simulink model "Zencar_rpo_2020_HIL_simulinkModel_PrebijaciStroj"  (R2020a)
settings: Solver=FixedStepAuto  StartTime=0.0  StopTime=150  FixedStep=1e-5  RelTol=1e-3
values from neighbouring files (symbols this model uses):
  b = 0.0002    [Zencar_rpo_2020_HIL_paramDef_PrebijaciStroj.m]
  cfi = 0.0137    [Zencar_rpo_2020_HIL_paramDef_PrebijaciStroj.m]
  g = 9.81    [Zencar_rpo_2020_HIL_paramDef_PrebijaciStroj.m]
  GR_overall = GR_rot*GR_transl    (= 0.000943396226415)    [Zencar_rpo_2020_HIL_paramDef_PrebijaciStroj.m]
  GR_rot = 1/53    (= 0.0188679245283)    [Zencar_rpo_2020_HIL_paramDef_PrebijaciStroj.m]
  GR_transl = 0.05    [Zencar_rpo_2020_HIL_paramDef_PrebijaciStroj.m]
  hal_maxi = 100    [Zencar_rpo_2020_HIL_paramDef_PrebijaciStroj.m]
  hal_maxv = 5    [Zencar_rpo_2020_HIL_paramDef_PrebijaciStroj.m]
  hal_zerov = 2.5    [Zencar_rpo_2020_HIL_paramDef_PrebijaciStroj.m]
  initial_pos = 0.25    [Zencar_rpo_2020_HIL_paramDef_PrebijaciStroj.m]
  J = J_motor+J_gearbox+J_endgear_and_press    (= 8.64998220007e-06)    [Zencar_rpo_2020_HIL_paramDef_PrebijaciStroj.m]
  K = k    [Zencar_rpo_2020_HIL_paramDef_PrebijaciStroj.m]
  La = 0.016e-3    (= 1.6e-05)    [Zencar_rpo_2020_HIL_paramDef_PrebijaciStroj.m]
  m_sys = 5    [Zencar_rpo_2020_HIL_paramDef_PrebijaciStroj.m]
  Nbar = Nu + K*Nx    [Zencar_rpo_2020_HIL_paramDef_PrebijaciStroj.m]
  Ra = 0.102    [Zencar_rpo_2020_HIL_paramDef_PrebijaciStroj.m]
  rot_enc_ppr = 2048    [Zencar_rpo_2020_HIL_paramDef_PrebijaciStroj.m]
  stroke = 0.3    [Zencar_rpo_2020_HIL_paramDef_PrebijaciStroj.m]
  Umax = 24    [Zencar_rpo_2020_HIL_paramDef_PrebijaciStroj.m]
settings Model: Creator=Palo  LastModifiedBy=Palo

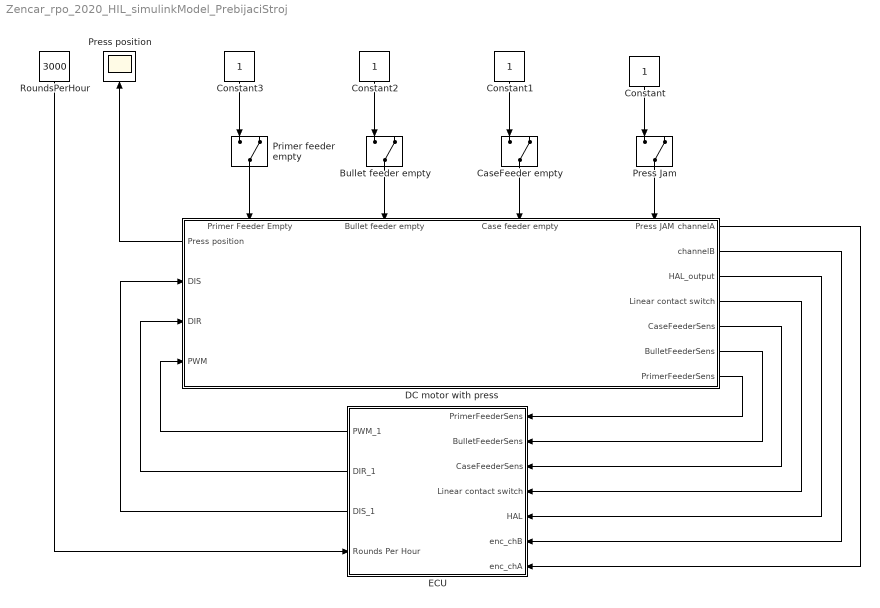
== system Zencar_rpo_2020_HIL_simulinkModel_PrebijaciStroj ==
  Bullet feeder empty : ManualSwitch  CurrentSetting=0
  CaseFeeder empty : ManualSwitch  CurrentSetting=0
  Constant{,1..3} (4 alike) : Constant
  DC motor with press : Subsystem
      settings: PortSchema="{\"entries\":[{\"content\":{\"sides\":[{\"content\":{\"connectorIds\":[\"Out8\",\"In1\",\"In2\",\"In3\"]},\"type\":\"ConnectorPlacement.EquallySpacedRectSide\",\"uuid\":\"44aa01d9-a270-4b10-8569-0796e281ce1b\"},{\"content\":{\"connectorIds\":[\"Out1\",\"Out2\",\"Out3\",\"Out4\",\"Out5\",\"Out6\",\"Out7\"],\"side\":\"RIGHT\"},\"type\":\"ConnectorPlacement.EquallySpacedRectSide\",\"uuid\":\"c8e5899d-1334-4fa1-8867-c03f8e90729c\"},{\"content\":{\"connectorIds\":[\"In4\",\"In5\",\"In6\",\"In7\"],\"side\":\"TOP\"},\"type\":\"ConnectorPlacement.EquallySpacedRectSide\",\"uuid\":\"b199ad83-4d3f-426f-a24f-893a662e75fe\"}]},\"type\":\"ConnectorPlacement.EquallySpacedConnector\",\"uuid\":\"598d06f8-804a-47b4-ba62-695d707896bf\"}],\"packageUris\":[\"http://schema.mathworks.com/mf0/Connector/19700101\"],\"version\":\"1.0\"}"
  ECU : Subsystem
      settings: PortSchema="{\"entries\":[{\"content\":{\"sides\":[{\"content\":{\"connectorIds\":[\"In1\",\"In2\",\"In3\",\"In4\",\"In5\",\"In6\",\"In7\"]},\"type\":\"ConnectorPlacement.EquallySpacedRectSide\",\"uuid\":\"89d60bc3-cc9c-43a7-ae0f-bebf81c284df\"},{\"content\":{\"connectorIds\":[\"Out1\",\"Out2\",\"Out3\",\"In8\"],\"side\":\"RIGHT\"},\"type\":\"ConnectorPlacement.EquallySpacedRectSide\",\"uuid\":\"e25504cb-4fdc-4ec0-83be-a621ed95c836\"},{\"content\":{\"connectorIds\":[],\"side\":\"TOP\"},\"type\":\"ConnectorPlacement.EquallySpacedRectSide\",\"uuid\":\"3fb693ce-24d4-4cc1-a1ce-0deb39646084\"}]},\"type\":\"ConnectorPlacement.EquallySpacedConnector\",\"uuid\":\"2bc13cae-35da-4195-ba30-c3443b14a144\"}],\"packageUris\":[\"http://schema.mathworks.com/mf0/Connector/19700101\"],\"version\":\"1.0\"}"
  Press Jam : ManualSwitch  CurrentSetting=0
  Press position : Scope
  Primer feeder empty : ManualSwitch  CurrentSetting=0
  RoundsPerHour : Constant  Value=3000
  wires:
  DC motor with press/1(channelA) -> ECU/7(enc_chA)
  DC motor with press/2(channelB) -> ECU/6(enc_chB)
  DC motor with press/3(HAL_output) -> ECU/5(HAL)
  ECU/1(PWM_1) -> DC motor with press/3(PWM)
  ECU/2(DIR_1) -> DC motor with press/2(DIR)
  ECU/3(DIS_1) -> DC motor with press/1(DIS)
  DC motor with press/4(Linear contact switch) -> ECU/4(Linear contact switch)
  Constant/1 -> Press Jam/1
  CaseFeeder empty/1 -> DC motor with press/6(Case feeder empty)
  Constant1/1 -> CaseFeeder empty/1
  Constant2/1 -> Bullet feeder empty/1
  DC motor with press/6(BulletFeederSens) -> ECU/2(BulletFeederSens)
  DC motor with press/5(CaseFeederSens) -> ECU/3(CaseFeederSens)
  Primer feeder empty/1 -> DC motor with press/4(Primer Feeder Empty)
  Constant3/1 -> Primer feeder empty/1
  DC motor with press/7(PrimerFeederSens) -> ECU/1(PrimerFeederSens)
  DC motor with press/8(Press position) -> Press position/1
  RoundsPerHour/1 -> ECU/8(Rounds Per Hour)
  Bullet feeder empty/1 -> DC motor with press/5(Bullet feeder empty)
  Press Jam/1 -> DC motor with press/7(Press JAM)

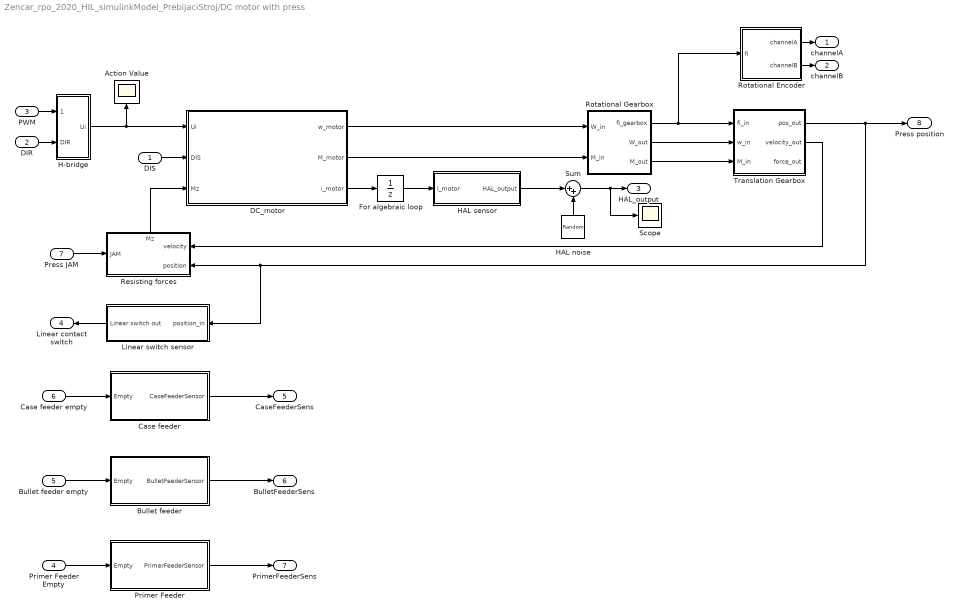
== system Zencar_rpo_2020_HIL_simulinkModel_PrebijaciStroj/DC motor with press ==
  DIS : Inport
  DIR : Inport  Port=2
  PWM : Inport  Port=3
  Primer Feeder Empty : Inport  Port=4
  Bullet feeder empty : Inport  Port=5
  Case feeder empty : Inport  Port=6
  Press JAM : Inport  Port=7
  Action Value : Scope
  Bullet feeder : Subsystem
  Case feeder : Subsystem
  DC_motor : Subsystem
  For algebraic loop : UnitDelay  SampleTime=-1  HasFrameUpgradeWarning=on
  H-bridge : Subsystem
  HAL noise : RandomNumber  Variance=3.3/10000  SampleTime=0.1
  HAL sensor : Subsystem
  Linear switch sensor : Subsystem
  Primer Feeder : Subsystem
  Resisting forces : Subsystem
      settings: PortSchema="{\"entries\":[{\"content\":{\"sides\":[{\"content\":{\"connectorIds\":[\"In1\"]},\"type\":\"ConnectorPlacement.EquallySpacedRectSide\",\"uuid\":\"f66e595a-d546-4368-bb4f-170145c9d05d\"},{\"content\":{\"connectorIds\":[\"In2\",\"In3\"],\"side\":\"RIGHT\"},\"type\":\"ConnectorPlacement.EquallySpacedRectSide\",\"uuid\":\"f401b9ee-f172-4854-b1a2-c293cdbafb20\"},{\"content\":{\"connectorIds\":[\"Out1\"],\"side\":\"TOP\"},\"type\":\"ConnectorPlacement.EquallySpacedRectSide\",\"uuid\":\"bb4b329b-5312-4992-9255-fed05c1ebbda\"}]},\"type\":\"ConnectorPlacement.EquallySpacedConnector\",\"uuid\":\"f4d49964-271c-4275-b048-9eeda0ea6065\"}],\"packageUris\":[\"http://schema.mathworks.com/mf0/Connector/19700101\"],\"version\":\"1.0\"}"
  Rotational Encoder : Subsystem
  Rotational Gearbox : Subsystem
  Scope : Scope
  Sum : Sum  Inputs=|++
  Translation Gearbox : Subsystem
  channelA : Outport
  channelB : Outport  Port=2
  HAL_output : Outport  Port=3
  Linear contact switch : Outport  Port=4
  CaseFeederSens : Outport  Port=5
  BulletFeederSens : Outport  Port=6
  PrimerFeederSens : Outport  Port=7
  Press position : Outport  Port=8
  wires:
  DC_motor/1(w_motor) -> Rotational Gearbox/1(W_in)
  DIR/1 -> H-bridge/2(DIR)
  Rotational Gearbox/2(W_out) -> Translation Gearbox/2(w_in)
  DC_motor/2(M_motor) -> Rotational Gearbox/2(M_in)
  H-bridge/1(Ui) -> DC_motor/1(Ui), Action Value/1
  Rotational Gearbox/3(M_out) -> Translation Gearbox/3(M_in)
  Rotational Encoder/2(channelB) -> channelB/1
  Rotational Encoder/1(channelA) -> channelA/1
  PWM/1 -> H-bridge/1(PWM)
  DC_motor/3(i_motor) -> For algebraic loop/1
  Rotational Gearbox/1(fi_gearbox) -> Rotational Encoder/1(fi), Translation Gearbox/1(fi_in)
  DIS/1 -> DC_motor/2(DIS)
  Translation Gearbox/1(pos_out) -> Press position/1, Resisting forces/3(position), Linear switch sensor/1(position_in)
  Translation Gearbox/2(velocity_out) -> Resisting forces/2(velocity)
  Linear switch sensor/1(Linear switch out) -> Linear contact switch/1
  Press JAM/1 -> Resisting forces/1(JAM)
  Case feeder empty/1 -> Case feeder/1(Empty)
  Bullet feeder empty/1 -> Bullet feeder/1(Empty)
  Bullet feeder/1(BulletFeederSensor) -> BulletFeederSens/1
  Case feeder/1(CaseFeederSensor) -> CaseFeederSens/1
  Primer Feeder/1(PrimerFeederSensor) -> PrimerFeederSens/1
  Primer Feeder Empty/1 -> Primer Feeder/1(Empty)
  For algebraic loop/1 -> HAL sensor/1(I_motor)
  HAL sensor/1(HAL_output) -> Sum/1
  Sum/1 -> Scope/1, HAL_output/1
  HAL noise/1 -> Sum/2
  Resisting forces/1(Mz) -> DC_motor/3(Mz)

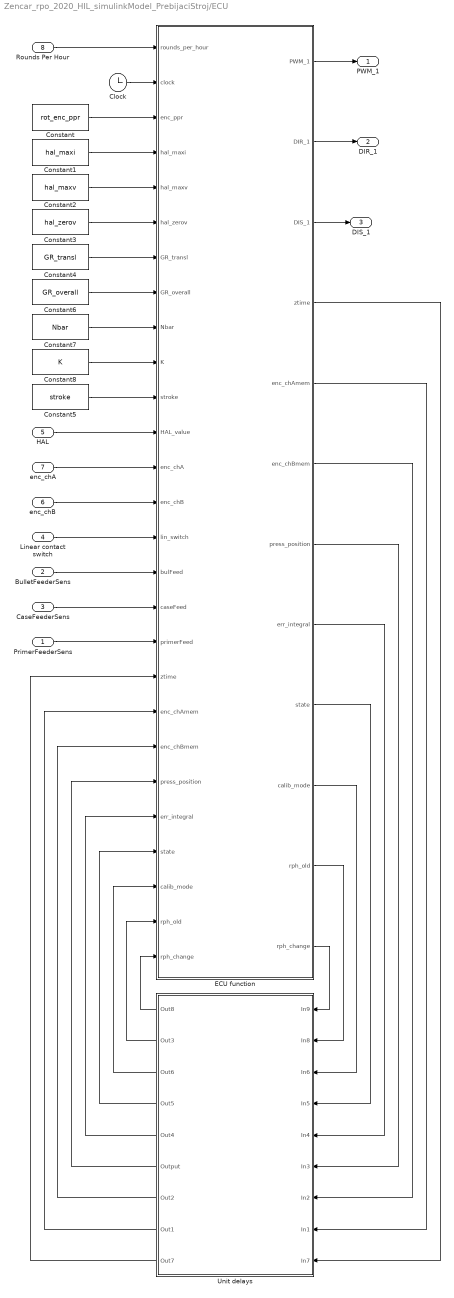
== system Zencar_rpo_2020_HIL_simulinkModel_PrebijaciStroj/ECU ==
  PrimerFeederSens : Inport
  BulletFeederSens : Inport  Port=2
  CaseFeederSens : Inport  Port=3
  Linear contact switch : Inport  Port=4
  HAL : Inport  Port=5
  enc_chB : Inport  Port=6
  enc_chA : Inport  Port=7
  Rounds Per Hour : Inport  Port=8
  Clock : Clock
  Constant : Constant  Value=rot_enc_ppr
  Constant1 : Constant  Value=hal_maxi
  Constant2 : Constant  Value=hal_maxv
  Constant3 : Constant  Value=hal_zerov
  Constant4 : Constant  Value=GR_transl
  Constant5 : Constant  Value=stroke
  Constant6 : Constant  Value=GR_overall
  Constant7 : Constant  Value=Nbar
  Constant8 : Constant  Value=K  VectorParams1D=off
  ECU function : MATLAB Function  TreatAsAtomicUnit=on
  Unit delays : Subsystem
  PWM_1 : Outport
  DIR_1 : Outport  Port=2
  DIS_1 : Outport  Port=3
  wires:
  enc_chA/1 -> ECU function/13(enc_chA)
  enc_chB/1 -> ECU function/14(enc_chB)
  ECU function/1(PWM_1) -> PWM_1/1
  ECU function/2(DIR_1) -> DIR_1/1
  Constant/1 -> ECU function/3(enc_ppr)
  HAL/1 -> ECU function/12(HAL_value)
  Constant1/1 -> ECU function/4(hal_maxi)
  Constant3/1 -> ECU function/6(hal_zerov)
  Constant2/1 -> ECU function/5(hal_maxv)
  ECU function/3(DIS_1) -> DIS_1/1
  Constant4/1 -> ECU function/7(GR_transl)
  Linear contact switch/1 -> ECU function/15(lin_switch)
  ECU function/5(enc_chAmem) -> Unit delays/8(In1)
  ECU function/6(enc_chBmem) -> Unit delays/7(In2)
  ECU function/8(err_integral) -> Unit delays/5(In4)
  Unit delays/8(Out1) -> ECU function/20("enc_chAmem ")
  Unit delays/7(Out2) -> ECU function/21("enc_chBmem ")
  Unit delays/6(Output) -> ECU function/22("press_position ")
  Unit delays/5(Out4) -> ECU function/23("err_integral ")
  ECU function/9(state) -> Unit delays/4(In5)
  ECU function/10(calib_mode) -> Unit delays/3(In6)
  Unit delays/4(Out5) -> ECU function/24("state ")
  Unit delays/3(Out6) -> ECU function/25("calib_mode ")
  Constant5/1 -> ECU function/11(stroke)
  Clock/1 -> ECU function/2(clock)
  Unit delays/9(Out7) -> ECU function/19("ztime ")
  ECU function/4(ztime) -> Unit delays/9(In7)
  BulletFeederSens/1 -> ECU function/16(bulFeed)
  CaseFeederSens/1 -> ECU function/17(caseFeed)
  PrimerFeederSens/1 -> ECU function/18(primerFeed)
  Unit delays/2(Out3) -> ECU function/26("rph_old ")
  ECU function/11(rph_old) -> Unit delays/2(In8)
  Unit delays/1(Out8) -> ECU function/27("rph_change ")
  ECU function/12(rph_change) -> Unit delays/1(In9)
  Rounds Per Hour/1 -> ECU function/1(rounds_per_hour)
  ECU function/7(press_position) -> Unit delays/6(In3)
  Constant6/1 -> ECU function/8(GR_overall)
  Constant7/1 -> ECU function/9(Nbar)
  Constant8/1 -> ECU function/10(K)

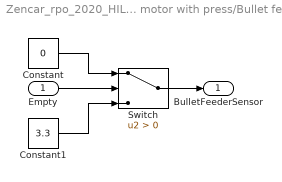
== system Zencar_rpo_2020_HIL_simulinkModel_PrebijaciStroj/DC motor with press/Bullet feeder ==
  Empty : Inport
  Constant : Constant  Value=0
  Constant1 : Constant  Value=3.3
  Switch : Switch  Criteria=u2 > Threshold
  BulletFeederSensor : Outport
  wires:
  Switch/1 -> BulletFeederSensor/1
  Constant1/1 -> Switch/3
  Constant/1 -> Switch/1
  Empty/1 -> Switch/2

== system Zencar_rpo_2020_HIL_simulinkModel_PrebijaciStroj/DC motor with press/Case feeder ==
  Empty : Inport
  Constant : Constant  Value=0
  Constant1 : Constant  Value=3.3
  Switch : Switch  Criteria=u2 > Threshold
  CaseFeederSensor : Outport
  wires:
  Empty/1 -> Switch/2
  Constant/1 -> Switch/1
  Constant1/1 -> Switch/3
  Switch/1 -> CaseFeederSensor/1

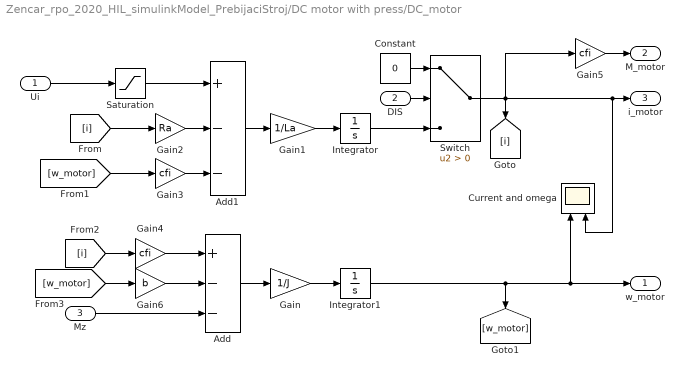
== system Zencar_rpo_2020_HIL_simulinkModel_PrebijaciStroj/DC motor with press/DC_motor ==
  Ui : Inport
  DIS : Inport  Port=2
  Mz : Inport  Port=3
  Add : Sum  Inputs=+--
  Add1 : Sum  Inputs=+--
  Constant : Constant  Value=0
  Current and omega : Scope  NumInputPorts=2
  Gain : Gain  Gain=1/J
  Gain1 : Gain  Gain=1/La
  Gain2 : Gain  Gain=Ra
  Gain3 : Gain  Gain=cfi
  Gain4 : Gain  Gain=cfi
  Gain5 : Gain  Gain=cfi
  Gain6 : Gain  Gain=b
  Integrator : Integrator
  Integrator1 : Integrator
  Saturation : Saturate  UpperLimit=Umax  LowerLimit=-Umax
  Switch : Switch  Criteria=u2 > Threshold
  w_motor : Outport
  M_motor : Outport  Port=2
  i_motor : Outport  Port=3
  wires:
  Add/1 -> Gain/1
  Gain/1 -> Integrator1/1
  Gain1/1 -> Integrator/1
  Add1/1 -> Gain1/1
  Gain2/1 -> Add1/2
  [i] -> Gain2/1
  [i] -> Gain4/1
  Gain3/1 -> Add1/3
  [w_motor] -> Gain3/1
  Gain4/1 -> Add/1
  Ui/1 -> Saturation/1
  Saturation/1 -> Add1/1
  Gain5/1 -> M_motor/1
  Integrator/1 -> Switch/3
  Switch/1 -> i_motor/1, Current and omega/2, Gain5/1, [i]
  DIS/1 -> Switch/2
  Constant/1 -> Switch/1
  Integrator1/1 -> Current and omega/1, w_motor/1, [w_motor]
  Mz/1 -> Add/3
  [w_motor] -> Gain6/1
  Gain6/1 -> Add/2

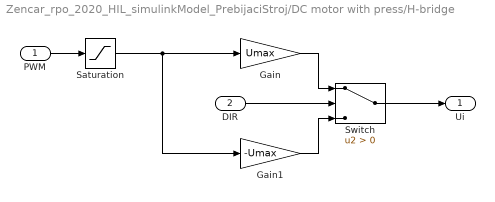
== system Zencar_rpo_2020_HIL_simulinkModel_PrebijaciStroj/DC motor with press/H-bridge ==
  PWM : Inport
  DIR : Inport  Port=2
  Gain : Gain  Gain=Umax
  Gain1 : Gain  Gain=-Umax
  Saturation : Saturate  UpperLimit=1  LowerLimit=0
  Switch : Switch  Criteria=u2 > Threshold
  Ui : Outport
  wires:
  DIR/1 -> Switch/2
  Gain/1 -> Switch/1
  PWM/1 -> Saturation/1
  Saturation/1 -> Gain1/1, Gain/1
  Gain1/1 -> Switch/3
  Switch/1 -> Ui/1

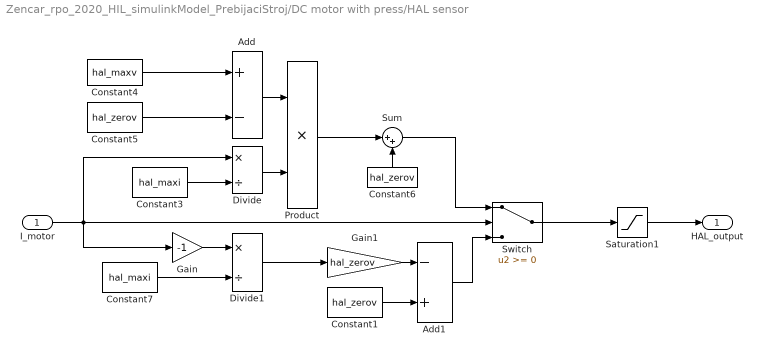
== system Zencar_rpo_2020_HIL_simulinkModel_PrebijaciStroj/DC motor with press/HAL sensor ==
  I_motor : Inport
  Add : Sum  Inputs=+-
  Add1 : Sum  Inputs=-+
  Constant1 : Constant  Value=hal_zerov
  Constant3 : Constant  Value=hal_maxi
  Constant4 : Constant  Value=hal_maxv
  Constant5 : Constant  Value=hal_zerov
  Constant6 : Constant  Value=hal_zerov
  Constant7 : Constant  Value=hal_maxi
  Divide : Product  Inputs=*/
  Divide1 : Product  Inputs=*/
  Gain : Gain  Gain=-1
  Gain1 : Gain  Gain=hal_zerov
  Product : Product
  Saturation1 : Saturate  UpperLimit=4.5  LowerLimit=0.5
  Sum : Sum  Inputs=|++
  Switch : Switch
  HAL_output : Outport
  wires:
  Constant4/1 -> Add/1
  Constant5/1 -> Add/2
  Add/1 -> Product/1
  Divide/1 -> Product/2
  Constant3/1 -> Divide/2
  Product/1 -> Sum/1
  Sum/1 -> Switch/1
  Constant6/1 -> Sum/2
  Gain/1 -> Divide1/1
  Constant7/1 -> Divide1/2
  Divide1/1 -> Gain1/1
  I_motor/1 -> Gain/1, Switch/2, Divide/1
  Gain1/1 -> Add1/1
  Add1/1 -> Switch/3
  Constant1/1 -> Add1/2
  Switch/1 -> Saturation1/1
  Saturation1/1 -> HAL_output/1

== system Zencar_rpo_2020_HIL_simulinkModel_PrebijaciStroj/DC motor with press/Linear switch sensor ==
  position_in : Inport
  Constant : Constant  Value=0
  Constant1 : Constant
  Switch : Switch  Threshold=stroke*0.25
  Linear switch out : Outport
  wires:
  position_in/1 -> Switch/2
  Constant/1 -> Switch/1
  Constant1/1 -> Switch/3
  Switch/1 -> Linear switch out/1

== system Zencar_rpo_2020_HIL_simulinkModel_PrebijaciStroj/DC motor with press/Primer Feeder ==
  Empty : Inport
  Constant : Constant  Value=0
  Constant1 : Constant  Value=3.3
  Switch : Switch  Criteria=u2 > Threshold
  PrimerFeederSensor : Outport
  wires:
  Switch/1 -> PrimerFeederSensor/1
  Constant1/1 -> Switch/3
  Constant/1 -> Switch/1
  Empty/1 -> Switch/2

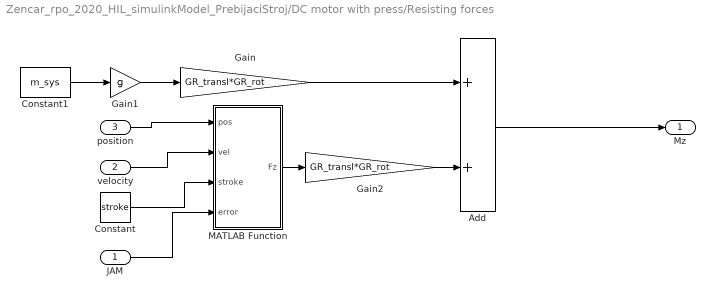
== system Zencar_rpo_2020_HIL_simulinkModel_PrebijaciStroj/DC motor with press/Resisting forces ==
  JAM : Inport
  velocity : Inport  Port=2
  position : Inport  Port=3
  Add : Sum
  Constant : Constant  Value=stroke
  Constant1 : Constant  Value=m_sys
  Gain : Gain  Gain=GR_transl*GR_rot
  Gain1 : Gain  Gain=g
  Gain2 : Gain  Gain=GR_transl*GR_rot
  MATLAB Function : MATLAB Function  TreatAsAtomicUnit=on
  Mz : Outport
  wires:
  Gain1/1 -> Gain/1
  Gain/1 -> Add/1
  Constant1/1 -> Gain1/1
  MATLAB Function/1(Fz) -> Gain2/1
  position/1 -> MATLAB Function/1(pos)
  velocity/1 -> MATLAB Function/2(vel)
  Constant/1 -> MATLAB Function/3(stroke)
  Add/1 -> Mz/1
  JAM/1 -> MATLAB Function/4(error)
  Gain2/1 -> Add/2

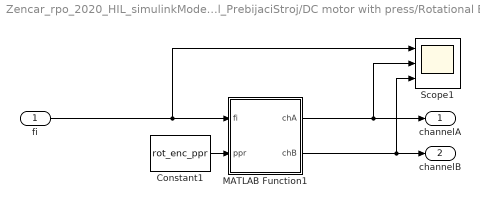
== system Zencar_rpo_2020_HIL_simulinkModel_PrebijaciStroj/DC motor with press/Rotational Encoder ==
  fi : Inport
  Constant1 : Constant  Value=rot_enc_ppr
  MATLAB Function1 : MATLAB Function  TreatAsAtomicUnit=on
  Scope1 : Scope  NumInputPorts=3
  channelA : Outport
  channelB : Outport  Port=2
  wires:
  MATLAB Function1/2(chB) -> channelB/1, Scope1/3
  Constant1/1 -> MATLAB Function1/2(ppr)
  MATLAB Function1/1(chA) -> channelA/1, Scope1/2
  fi/1 -> Scope1/1, MATLAB Function1/1(fi)

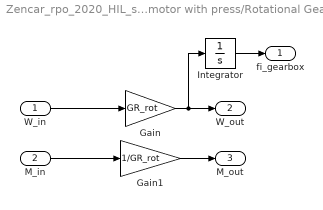
== system Zencar_rpo_2020_HIL_simulinkModel_PrebijaciStroj/DC motor with press/Rotational Gearbox ==
  W_in : Inport
  M_in : Inport  Port=2
  Gain : Gain  Gain=GR_rot
  Gain1 : Gain  Gain=1/GR_rot
  Integrator : Integrator  InitialCondition=initial_pos/GR_transl
  fi_gearbox : Outport
  W_out : Outport  Port=2
  M_out : Outport  Port=3
  wires:
  W_in/1 -> Gain/1
  M_in/1 -> Gain1/1
  Gain/1 -> Integrator/1, W_out/1
  Gain1/1 -> M_out/1
  Integrator/1 -> fi_gearbox/1

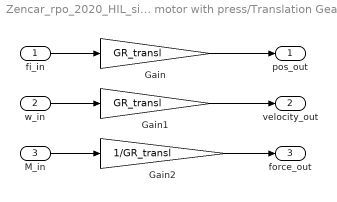
== system Zencar_rpo_2020_HIL_simulinkModel_PrebijaciStroj/DC motor with press/Translation Gearbox ==
  fi_in : Inport
  w_in : Inport  Port=2
  M_in : Inport  Port=3
  Gain : Gain  Gain=GR_transl
  Gain1 : Gain  Gain=GR_transl
  Gain2 : Gain  Gain=1/GR_transl
  pos_out : Outport
  velocity_out : Outport  Port=2
  force_out : Outport  Port=3
  wires:
  fi_in/1 -> Gain/1
  Gain/1 -> pos_out/1
  Gain1/1 -> velocity_out/1
  w_in/1 -> Gain1/1
  M_in/1 -> Gain2/1
  Gain2/1 -> force_out/1

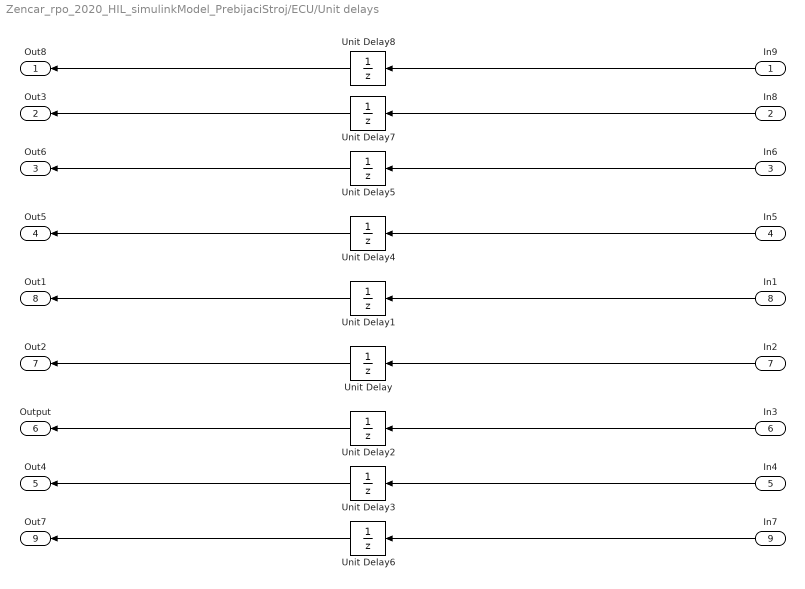
== system Zencar_rpo_2020_HIL_simulinkModel_PrebijaciStroj/ECU/Unit delays ==
  In9 : Inport
  In8 : Inport  Port=2
  In6 : Inport  Port=3
  In5 : Inport  Port=4
  In4 : Inport  Port=5
  In3 : Inport  Port=6
  In2 : Inport  Port=7
  In1 : Inport  Port=8
  In7 : Inport  Port=9
  Unit Delay{,1..8} (9 alike) : UnitDelay  SampleTime=-1  HasFrameUpgradeWarning=on
  Out8 : Outport
  Out3 : Outport  Port=2
  Out6 : Outport  Port=3
  Out5 : Outport  Port=4
  Out4 : Outport  Port=5
  Output : Outport  Port=6
  Out2 : Outport  Port=7
  Out1 : Outport  Port=8
  Out7 : Outport  Port=9
  wires:
  Unit Delay/1 -> Out2/1
  Unit Delay3/1 -> Out4/1
  Unit Delay2/1 -> Output/1
  In4/1 -> Unit Delay3/1
  In2/1 -> Unit Delay/1
  In3/1 -> Unit Delay2/1
  Unit Delay1/1 -> Out1/1
  In1/1 -> Unit Delay1/1
  In5/1 -> Unit Delay4/1
  Unit Delay5/1 -> Out6/1
  In6/1 -> Unit Delay5/1
  Unit Delay4/1 -> Out5/1
  In7/1 -> Unit Delay6/1
  Unit Delay6/1 -> Out7/1
  In8/1 -> Unit Delay7/1
  Unit Delay7/1 -> Out3/1
  In9/1 -> Unit Delay8/1
  Unit Delay8/1 -> Out8/1

== matlab function Zencar_rpo_2020_HIL_simulinkModel_PrebijaciStroj/DC motor with press/Rotational Encoder/MATLAB Function1 ==
  data: fi input; chA output; ppr input; chB output
function [chA,chB] = fcn(fi,ppr)

%clockwise direction - channel B before channel A
%anticlockwise direction - channel A before channel B

per=2*pi/ppr;%period
hper=per/2;%half period
qper=per/4;%quarter period

%channel A
zeroedFi=fi - (floor(fi/per)*per);
chA=floor(zeroedFi/hper);


%channel B
zeroedFi=fi - (floor(fi/per)*per) - qper;
if(zeroedFi<=hper &  zeroedFi>0)
    chB=1;
else
    chB=0;
end













% if(zeroedFi<=hper)
%     chA=0;
% else
%     chA=1;
% end

== matlab function Zencar_rpo_2020_HIL_simulinkModel_PrebijaciStroj/DC motor with press/Resisting forces/MATLAB Function ==
  data: pos input; Fz output; vel input; stroke input; error input
function Fz = fcn(pos,vel,stroke,error)
Fz=0;
if(vel>=0)
    if(pos > stroke*0.8)
       Fz=300; 
    else
        Fz=0;
    end
    
    if(error==1 & pos>stroke*0.9)
        Fz=15000;
    end 
    
    if(pos>stroke+0.01)
        Fz=15000;
    end
end
if(vel<0)
    if(pos<stroke*0.1)
        Fz=-150;
    else
        Fz=0;
    end
    
    if(pos>stroke*0.8)
        Fz=-150;
    end
    
    if(pos<-0.01)
        Fz=-9000;
    end
end

== matlab function Zencar_rpo_2020_HIL_simulinkModel_PrebijaciStroj/ECU/ECU function ==
  data: PWM_1 output; DIR_1 output; DIS_1 output; ztime output; enc_chAmem output; enc_chBmem output; press_position output; rounds_per_hour input; clock input; enc_ppr input; hal_maxi input; hal_maxv input; hal_zerov input; GR_transl input; GR_overall input; Nbar input; K input; stroke input; HAL_value input; enc_chA input; enc_chB input; lin_switch input; bulFeed input; caseFeed input; primerFeed input; ztime input; enc_chAmem input; enc_chBmem input; press_position input; err_integral input; err_integral output; state input; state output; calib_mode input; calib_mode output; rph_old output; rph_old input; rph_change output; rph_change input
function [PWM_1,DIR_1,DIS_1,ztime, enc_chAmem,enc_chBmem,press_position,err_integral,state, calib_mode, rph_old, rph_change] = fcn(rounds_per_hour, clock, enc_ppr,hal_maxi,hal_maxv,hal_zerov,GR_transl,GR_overall, Nbar, K, stroke, HAL_value,enc_chA,enc_chB,lin_switch,bulFeed, caseFeed, primerFeed, ztime, enc_chAmem,enc_chBmem,press_position,err_integral,state,calib_mode, rph_old, rph_change)
%%
PWM_1=0;
DIR_1=0;
DIS_1=0;

dfi=0;
wanted_position=0;

%HALL decoding
if(HAL_value>=hal_zerov)
    motor_i=(HAL_value-hal_zerov)/(hal_maxv-hal_zerov)*hal_maxi;
elseif(HAL_value<hal_zerov)
    motor_i=-(hal_zerov-HAL_value)/hal_zerov*hal_maxi;
else
    motor_i=0;
end

%encoder decoding 
if(enc_chAmem==1 & enc_chBmem==1)
   if(enc_chA==1 & enc_chB==0)
       dfi=2*pi/(4*enc_ppr);
   end
   if(enc_chA==0 & enc_chB==1)
       dfi=-2*pi/(4*enc_ppr);
   end
end

if(enc_chAmem==0 & enc_chBmem==0)
   if(enc_chA==0 & enc_chB==1)
       dfi=2*pi/(4*enc_ppr);
   end
   if(enc_chA==1 & enc_chB==0)
       dfi=-2*pi/(4*enc_ppr);
   end
end

if(enc_chAmem==0 & enc_chBmem==1)
    if(enc_chA==1 & enc_chB==1)
        dfi=+2*pi/(4*enc_ppr);
    end
    if(enc_chA==0 & enc_chB==0)
        dfi=-2*pi/(4*enc_ppr);
    end
end

if(enc_chAmem==1 & enc_chBmem==0)
    if(enc_chA==1 & enc_chB==1)
        dfi=-2*pi/(4*enc_ppr);
    end
    if(enc_chA==0 & enc_chB==0)
        dfi=+2*pi/(4*enc_ppr);
    end
end
enc_chAmem=enc_chA;
enc_chBmem=enc_chB;
press_position=press_position+dfi*GR_transl;

%% Check errors

if(abs(motor_i) > 60)
    state=3;%overcurrent error
end

if(dfi>0 & press_position>=stroke*0.1 & press_position<=stroke*0.11)
    if(bulFeed~=3.3 | caseFeed~=3.3 | primerFeed~=3.3)
        state=4;%bullet feeder empty or casefeeder empty or bullet feeder die malfunction or primer feeder empty
    end
end




switch(state)
    case 0
        if(calib_mode==0)
            if lin_switch==0
                calib_mode=1;
            else
                calib_mode=2;
            end
        end
        if(calib_mode==1)
                if(lin_switch==1)
                    press_position=stroke*0.25;
                    state=1;
                    return
                end
                PWM_1=0.05;
                DIR_1=0;
        end
            
        if(calib_mode==2)
                if(lin_switch==0)
                    press_position=stroke*0.25;
                    state=1;
                    return
                end
                PWM_1=0.05;
                DIR_1=1;
        end
    case 1
        if(press_position>0)
            PWM_1=0.05;
            DIR_1=0;
        else
            state=2;
            ztime=clock;
        end
    case 2
        %% Regulator
        if(rounds_per_hour~=rph_old & rph_change==0)
            rph_change=1;
        end
        %changing working frequency only in the bottom position
        if(rph_change==1 & press_position<=5e-4)
            work_freq=rounds_per_hour*(2*pi)/3600;
            rph_change=0;
            rph_old=rounds_per_hour;
            ztime=clock;
        elseif(rph_change==1 & press_position>5e-4)
            work_freq=rph_old*(2*pi)/3600;
        else
            work_freq=rounds_per_hour*(2*pi)/3600;
            rph_old=rounds_per_hour;
        end
                   
        wanted_position=0.999*(stroke/2)*sin(work_freq*(clock-ztime)-pi/2)+0.999*(stroke/2);
        
        %P regulator
%         P=3000;
%         pos_error=wanted_position-press_position;    
%         PWM_1=P*pos_error;

        
        %LQR regulator
        LQR_wanted_pos = wanted_position * Nbar / GR_overall;    
        PWM_1= - K*[press_position/GR_overall 0 motor_i]' + LQR_wanted_pos;
        


        %PWM generation
        if(PWM_1>24)
            PWM_1=24;
        elseif(PWM_1<-24)
            PWM_1=-24;
        else
            PWM_1=PWM_1;
        end

        if(PWM_1>=0)
            DIR_1=1;
        else
            DIR_1=0;
        end
        PWM_1=abs(PWM_1)/24;
    case 3
        %% Error
        wanted_position=stroke*0.9-0.05;
        LQR_wanted_pos = wanted_position * Nbar / GR_overall;
        
        PWM_1= - K*[press_position/GR_overall 0 motor_i]' + LQR_wanted_pos;
        


        %PWM generation
        if(PWM_1>24)
            PWM_1=24;
        elseif(PWM_1<-24)
            PWM_1=-24;
        else
            PWM_1=PWM_1;
        end

        if(PWM_1>=0)
            DIR_1=1;
        else
            DIR_1=0;
        end
        PWM_1=abs(PWM_1)/24;
    case 4
        %% Error
        PWM_1=0;
        DIR_1=0;
        if(bulFeed==3.3 & caseFeed==3.3 & primerFeed)
            state=1;
        end
        
end
